simulink model "system_blocks_carsim"  (Simulink 10.0)
settings: Solver=ode45  StartTime=0  StopTime=10  FixedStep=0.002  RelTol=1e-3  AbsTol=1e-6
libraries: Solver_SF x1, mpclib x1
settings Model: Creator=ywata  LastModifiedBy=Vish  ExtModeTrigMode=oneshot  ExtModeArmWhenConnect=off
settings SolverCC: AutoScaleAbsTol=off
settings DataIOCC: SignalLoggingSaveFormat=ModelDataLogs  SignalLoggingName=sigsOut
settings OptimizationCC: BooleanDataType=off  ExpressionDepthLimit=2147483647
settings DebuggingCC: SaveWithParameterizedLinksMsg=none  SignalResolutionControl=TryResolveAllWithWarning  MultiTaskDSMMsg=warning  MultiTaskCondExecSysMsg=none  FcnCallInpInsideContextMsg=warning  StateNameClashWarn=warning
settings HardwareCC: TargetUnknown=on
settings RTWCC: TemplateMakefile=grt_vc.tmf
settings GRTTargetCC: GeneratePreprocessorConditionals=Disable all
settings ConfigComp: CovExternalEMLEnable=off

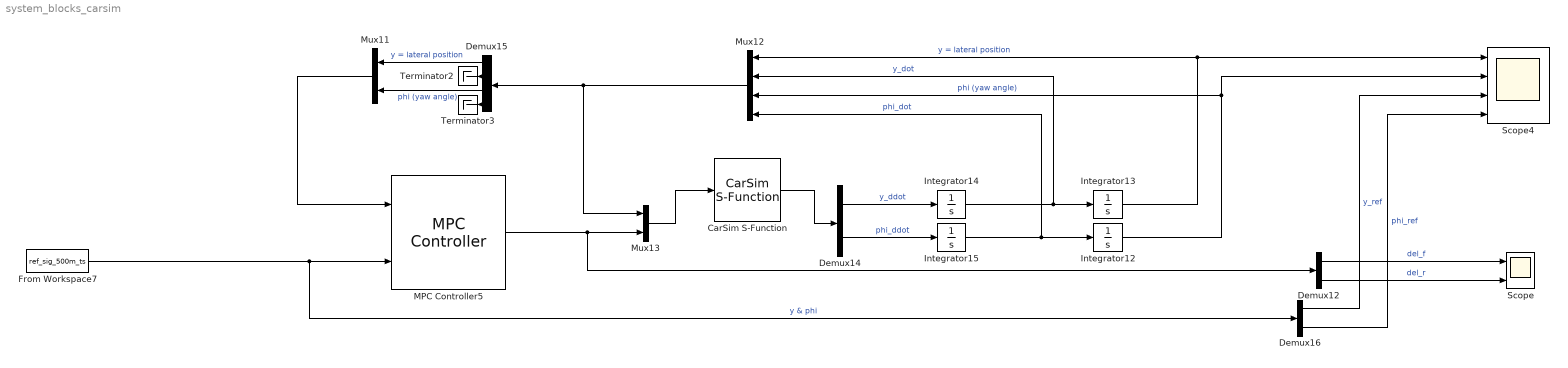
== system system_blocks_carsim ==
  CarSim S-Function : Solver_SF/CarSim S-Function  Priority=1  SIMFILE=simfile.sim
  Demux12 : Demux  Outputs=2
  Demux14 : Demux  Outputs=2
  Demux15 : Demux
  Demux16 : Demux  Outputs=2
  From Workspace7 : FromWorkspace  VariableName=ref_sig_500m_ts  SampleTime=0
  Integrator{12..15} (4 alike) : Integrator
  MPC Controller5 : mpclib/MPC Controller  SCDEnableBlockLinearizationSpecification=on  mpcobj=mpc1  is_multiple=0  enable_value=0  return_u0=off  updateMPCinCallerWorkspace=on  md_inport=off  mv_inport=off  uref_inport=off  return_cost=off  return_mvseq=off  return_qpstatus=off  return_xseq=off  return_state=off  return_ovseq=off  state_inport=off  umin_inport=off  umax_inport=off  ymin_inport=off  ymax_inport=off  cc_inport=off  ywt_inport=off  uwt_inport=off  duwt_inport=off  rhoeps_inport=off  pm_inport=off  MaximumP=10  HorizonChoice=FixedHorizon  n_ts=0.1  n_p=15  n_mv=2  n_md=0  n_ud=0  n_mo=2  n_uo=0  BlockDataType=double  SampleTimeInherited=off  switch_inport=off
  Mux11 : Mux  Inputs=2
  Mux12 : Mux
  Mux13 : Mux  Inputs=2
  Scope : Scope  NumInputPorts=2
  Scope4 : Scope  NumInputPorts=4
  Terminator2 : Terminator
  Terminator3 : Terminator
  wires:
  Mux13/1 -> CarSim S-Function/1
  From Workspace7/1 -> MPC Controller5/2, Demux16/1  "y & phi"
  Demux15/3 -> Mux11/2  "phi (yaw angle)"
  Demux15/1 -> Mux11/1  "y = lateral position"
  Integrator14/1 -> Mux12/2, Integrator13/1  "y_dot"
  Demux14/2 -> Integrator15/1  "phi_ddot"
  Mux11/1 -> MPC Controller5/1
  Demux12/2 -> Scope/2  "del_r"
  Demux16/2 -> Scope4/4  "phi_ref"
  Integrator13/1 -> Mux12/1, Scope4/1  "y = lateral position"
  Demux14/1 -> Integrator14/1  "y_ddot"
  Demux16/1 -> Scope4/3  "y_ref"
  Demux15/2 -> Terminator2/1
  Integrator12/1 -> Scope4/2, Mux12/3  "phi (yaw angle)"
  Demux15/4 -> Terminator3/1
  Demux12/1 -> Scope/1  "del_f"
  Integrator15/1 -> Mux12/4, Integrator12/1  "phi_dot"
  MPC Controller5/1 -> Demux12/1, Mux13/2
  Mux12/1 -> Demux15/1, Mux13/1
  CarSim S-Function/1 -> Demux14/1
